simulink model "Lab1_mdl_diskr"  (R2013b)
settings: Solver=ode3  StartTime=0.0  StopTime=100.0  FixedStep=10e-3  RelTol=1e-3
undefined symbols (not defined in the file or in its folder): Ad, Bd, Cd
settings Model: Creator=user  LastModifiedBy=user
settings DataIOCC: LimitDataPoints=off

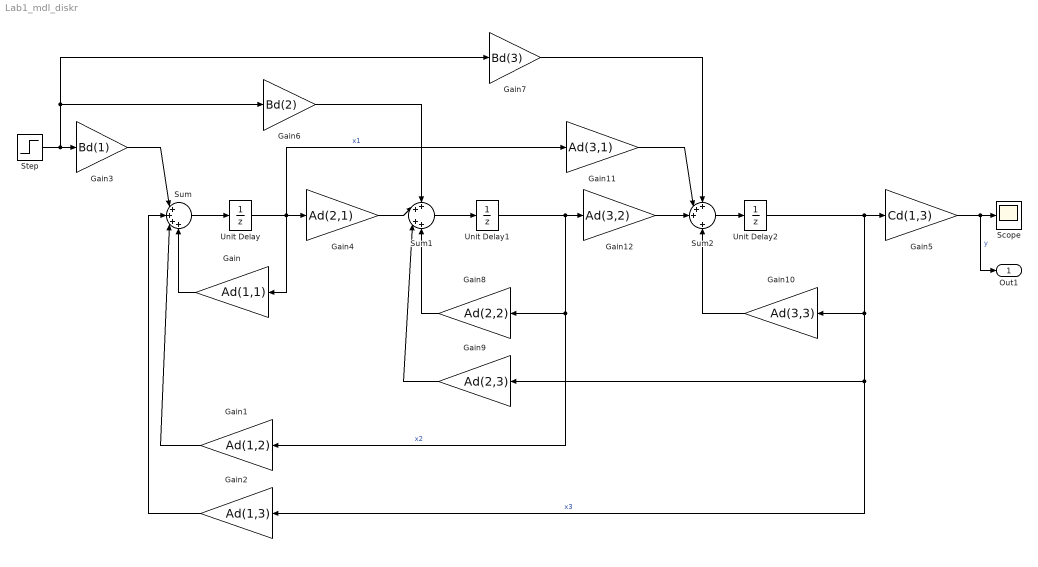
== system Lab1_mdl_diskr ==
  Gain : Gain  Gain=Ad(1,1)
  Gain1 : Gain  Gain=Ad(1,2)
  Gain10 : Gain  Gain=Ad(3,3)
  Gain11 : Gain  Gain=Ad(3,1)
  Gain12 : Gain  Gain=Ad(3,2)
  Gain2 : Gain  Gain=Ad(1,3)
  Gain3 : Gain  Gain=Bd(1)
  Gain4 : Gain  Gain=Ad(2,1)
  Gain5 : Gain  Gain=Cd(1,3)
  Gain6 : Gain  Gain=Bd(2)
  Gain7 : Gain  Gain=Bd(3)
  Gain8 : Gain  Gain=Ad(2,2)
  Gain9 : Gain  Gain=Ad(2,3)
  Scope : Scope
      settings: SaveName=DiscrMdl
  Step : Step  Time=0  SampleTime=0.4  mask(DiscretizedSource){}
      mask init:
      | %zoh
  Sum : Sum  Inputs=|++++
  Sum1 : Sum  Inputs=++|++
  Sum2 : Sum  Inputs=+++|+
  Unit Delay : UnitDelay  SampleTime=0.4
  Unit Delay1 : UnitDelay  SampleTime=0.4
  Unit Delay2 : UnitDelay  SampleTime=0.4
  Out1 : Outport
  wires:
  Unit Delay/1 -> Gain11/1, Gain4/1, Gain/1  "x1"
  Sum/1 -> Unit Delay/1
  Gain/1 -> Sum/4
  Gain1/1 -> Sum/3
  Gain2/1 -> Sum/2
  Gain3/1 -> Sum/1
  Step/1 -> Gain6/1, Gain7/1, Gain3/1
  Gain5/1 -> Out1/1, Scope/1  "y"
  Gain4/1 -> Sum1/2
  Sum1/1 -> Unit Delay1/1
  Gain6/1 -> Sum1/1
  Sum2/1 -> Unit Delay2/1
  Gain7/1 -> Sum2/1
  Unit Delay1/1 -> Gain8/1, Gain1/1, Gain12/1  "x2"
  Gain8/1 -> Sum1/4
  Gain9/1 -> Sum1/3
  Unit Delay2/1 -> Gain5/1, Gain9/1, Gain2/1, Gain10/1  "x3"
  Gain12/1 -> Sum2/3
  Gain10/1 -> Sum2/4
  Gain11/1 -> Sum2/2
